simulink model "quadSim"  (R2019a)
settings: Solver=ode45  StartTime=0.0  StopTime=20  MaxStep=0.001  RelTol=1e-6  EnableMultiTasking=on
values from neighbouring files (symbols this model uses):
  bodyHalf = 0.3    [drone.m]
  hoverVel = trustPerPropeller / Ktrust    (= 50.511573882)    [drone.m]
  hoverVoltage = hoverCurrent * Ra + hoverRPM / Kv    (= 1.1)    [drone.m]
  KDrag = ampMax * Km / (rpmMax / 60 * 2 * pi)    (= 7.30185461146e-05)    [drone.m]    (also in propeller.m = 5.03149938834e-05)
  Km = 60/(Kv * 2 * pi)    (= 0.00536477336265)    [drone.m]    (also in propeller.m)
  Ktrust = (trustMax * g)/(rpmMax / 60 * 2 * pi)    (= 0.0427122505634)    [drone.m]    (also in propeller.m = 0.00501338070739)
  motorMass = 0.055    [drone.m]
  propellerMass = 0.015    [drone.m]
  Ra = RaVolt/ampMax    (= 1.20584269663)    [drone.m]    (also in propeller.m = 0.173442288049)
  s = tf('s')    [step-af-drone.m]
  Ts = 0.002    [drone.m]    (also in propeller.m)
undefined symbols (not defined in the file or in its folder): X, Y, Z
libraries: sm_lib x32, nesl_utility x23
(part 1 of 2)
settings Model: Creator=chr  LastModifiedBy=Hillerup
settings DataIOCC: LimitDataPoints=on  SaveFormat=Array  ReturnWorkspaceOutputs=off
settings OptimizationCC: LifeSpan=inf
settings DebuggingCC: SFUnexpectedBacktrackingDiag=warning  SFNoUnconditionalDefaultTransitionDiag=warning  SFExecutionAtInitializationDiag=none  ArithmeticOperatorsInVariantConditions=warning
settings HardwareCC: ProdBitPerPointer=32  ProdBitPerSizeT=32  ProdBitPerPtrDiffT=32  ProdLargestAtomicFloat=None  ProdIntDivRoundTo=Undefined  ProdEndianess=Unspecified  ProdWordSize=32  ProdHWDeviceType=32-bit Generic
settings ModelReferenceCC: PropagateSignalLabelsOutOfModel=off
settings SFSimCC: SimUseLocalCustomCode=off
settings RTWCC: RTWUseLocalCustomCode=off
settings CodeAppCC: StateflowObjectComments=on
settings GRTTargetCC: TargetLangStandard=C89/C90 (ANSI)  GeneratePreprocessorConditionals=Disable all
settings ConfigComp: CovMetricSettings=dw  CovHtmlReporting=on  CovSaveCumulativeToWorkspaceVar=on  CovSaveSingleToWorkspaceVar=on  CovExternalEMLEnable=off
settings SimscapeCC: SimscapeNormalizeSystem=off  SimscapeLogType=all  SimscapeLogDataHistory=10000
settings ConfigurationSet: Description=SimMechanics 2G

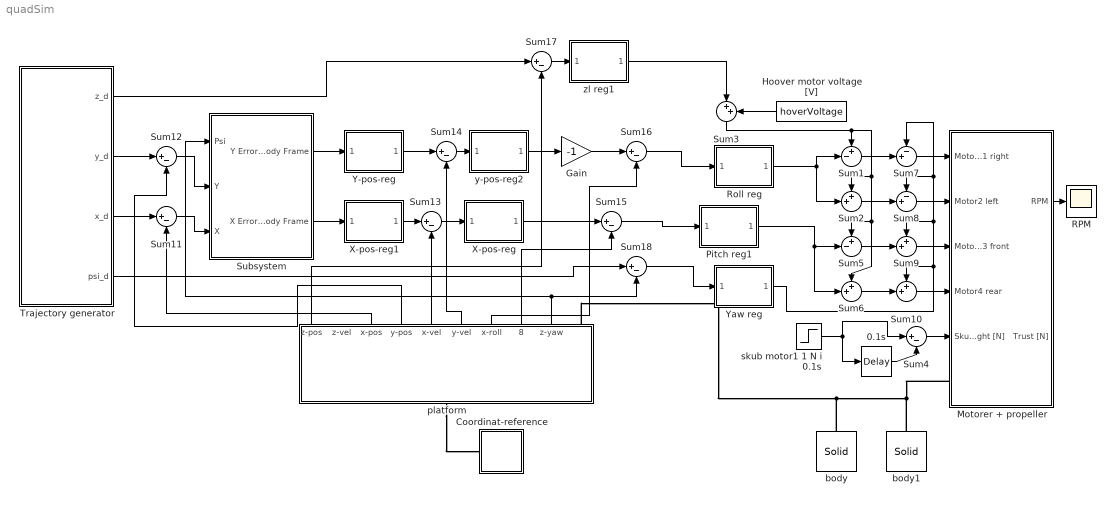
== system quadSim ==
  0.1s : TransportDelay  DelayTime=0.1
  Coordinat-reference : Subsystem
  Gain : Gain  Gain=-1
  Hoover motor voltage [V] : Constant  Value=hoverVoltage
  Motorer + propeller : Subsystem
  Pitch reg1 : Subsystem
  RPM : Scope
  Roll reg : Subsystem
  Subsystem : Subsystem
  Sum1 : Sum  Inputs=+-|
  Sum{2,6,9..10} (4 alike) : Sum  Inputs=++|
  Sum{4,11..18} (9 alike) : Sum  Inputs=|+-
  Sum3 : Sum  Inputs=|++
  Sum5 : Sum  Inputs=+-|
  Sum7 : Sum  Inputs=-+|
  Sum8 : Sum  Inputs=-+|
  Trajectory generator : Subsystem  TreatAsAtomicUnit=on
  X-pos-reg : Subsystem
  X-pos-reg1 : Subsystem
  Y-pos-reg : Subsystem
  "Yaw reg " : Subsystem
  body : sm_lib/Body Elements/Solid  InertiaType=CalculateFromGeometry  Mass=bodyHalf  MassUnits=kg  CenterOfMass=[0 0 0]  CenterOfMassUnits=m  MomentsOfInertia=[1 1 1]  MomentsOfInertiaUnits=kg*m^2  ProductsOfInertia=[0 0 0]  ProductsOfInertiaUnits=kg*m^2  BasedOnType=Mass  Density=1000  DensityUnits=kg/(m^3)  DoExposeReferenceFrame=on  SerializedFrames=<Frames/>  GraphicType=FromGeometry  MarkerShape=Sphere  MarkerSize=10  MarkerSizeUnits=m  GraphicVisPropType=SimpleVisualProperties  GraphicDiffuseColor=[0.5 0.5 0.5]  GraphicSpecularColor=[0.5 0.5 0.5 1.0]  GraphicAmbientColor=[0.15 0.15 0.15 1.0]  GraphicEmissiveColor=[0.0 0.0 0.0 1.0]  GraphicShininess=75  GraphicOpacity=1.0  GeometryShape=Brick  RectangleSize=[1 1]  RectangleSizeUnits=m  BrickDimensions=[0.04 0.4 0.03]  BrickDimensionUnits=m  CylinderRadius=0.02  CylinderRadiusUnits=m  CylinderLength=0.05  CylinderLengthUnits=m  SphereRadius=1  SphereRadiusUnits=m  EllipsoidRadii=[1 1 1]  EllipsoidRadiiUnits=m  ExtrusionCrossSection=[1 1; -1 1; -1 -1; 1 -1]  ExtrusionCrossSectionUnits=m  ExtrusionLength=1  ExtrusionLengthUnits=m  PolygonNumSides=3  PolygonOuterRadius=1  PolygonOuterRadiusUnits=m  ExtGeomFileType=STL  ExtGeomFileUnits=m  RevolutionCrossSection=[1 1; 1 -1; 2 -1; 2 1]  RevolutionCrossSectionUnits=m  RevolutionExtent=Full  RevolutionAngle=180  RevolutionAngleUnits=deg
  body1 : sm_lib/Body Elements/Solid  InertiaType=CalculateFromGeometry  Mass=bodyHalf  MassUnits=kg  CenterOfMass=[0 0 0]  CenterOfMassUnits=m  MomentsOfInertia=[1 1 1]  MomentsOfInertiaUnits=kg*m^2  ProductsOfInertia=[0 0 0]  ProductsOfInertiaUnits=kg*m^2  BasedOnType=Mass  Density=1000  DensityUnits=kg/(m^3)  DoExposeReferenceFrame=on  SerializedFrames=<Frames/>  GraphicType=FromGeometry  MarkerShape=Sphere  MarkerSize=10  MarkerSizeUnits=m  GraphicVisPropType=SimpleVisualProperties  GraphicDiffuseColor=[0.5 0.5 0.5]  GraphicSpecularColor=[0.5 0.5 0.5 1.0]  GraphicAmbientColor=[0.15 0.15 0.15 1.0]  GraphicEmissiveColor=[0.0 0.0 0.0 1.0]  GraphicShininess=75  GraphicOpacity=1.0  GeometryShape=Brick  RectangleSize=[1 1]  RectangleSizeUnits=m  BrickDimensions=[0.4 0.04 0.03]  BrickDimensionUnits=m  CylinderRadius=0.02  CylinderRadiusUnits=m  CylinderLength=0.05  CylinderLengthUnits=m  SphereRadius=1  SphereRadiusUnits=m  EllipsoidRadii=[1 1 1]  EllipsoidRadiiUnits=m  ExtrusionCrossSection=[1 1; -1 1; -1 -1; 1 -1]  ExtrusionCrossSectionUnits=m  ExtrusionLength=1  ExtrusionLengthUnits=m  PolygonNumSides=3  PolygonOuterRadius=1  PolygonOuterRadiusUnits=m  ExtGeomFileType=STL  ExtGeomFileUnits=m  RevolutionCrossSection=[1 1; 1 -1; 2 -1; 2 1]  RevolutionCrossSectionUnits=m  RevolutionExtent=Full  RevolutionAngle=180  RevolutionAngleUnits=deg
  platform : Subsystem
  skub motor1 1 N i 0.1s : Step  Time=2  SampleTime=0
  y-pos-reg2 : Subsystem
  zl reg1 : Subsystem
  wires:
  Motorer + propeller/1(RPM) -> RPM/1
  Sum3/1 -> Sum1/1, Sum6/1, Sum5/1, Sum2/1
  Sum4/1 -> Motorer + propeller/5(Skub right [N])
  Sum1/1 -> Sum7/2
  Sum2/1 -> Sum8/2
  Sum5/1 -> Sum9/2
  Sum6/1 -> Sum10/2
  Sum10/1 -> Motorer + propeller/4(Motor4 rear)
  Sum9/1 -> Motorer + propeller/3(Motor3 front)
  Sum8/1 -> Motorer + propeller/2(Motor2 left)
  Sum7/1 -> Motorer + propeller/1(Motor1 right)
  skub motor1 1 N i 0.1s/1 -> Sum4/1, 0.1s/1
  0.1s/1 -> Sum4/2
  platform/9(z-yaw) -> Sum18/2, Subsystem/1(Psi)
  Hoover motor voltage [V]/1 -> Sum3/2
  platform/3(x-pos) -> Sum11/2
  Trajectory generator/3(x_d) -> Sum11/1
  Sum11/1 -> Subsystem/3(X)
  Sum12/1 -> Subsystem/2(Y)
  Trajectory generator/2(y_d) -> Sum12/1
  zl reg1/1(u-roll) -> Sum3/1
  "Yaw reg "/1(u - yaw) -> Sum7/1, Sum8/1, Sum9/1, Sum10/1
  platform/7(x-roll) -> Sum16/2
  Sum17/1 -> zl reg1/1(error)
  Trajectory generator/1(z_d) -> Sum17/1
  platform/1(z-pos) -> Sum17/2
  Sum15/1 -> Pitch reg1/1(error)
  Sum18/1 -> "Yaw reg "/1(error)
  Trajectory generator/4(psi_d) -> Sum18/1
  platform/8(y-pitch) -> Sum15/2
  Subsystem/1(Y Error in Body Frame) -> Y-pos-reg/1(error_y)
  Subsystem/2(X Error in body Frame) -> X-pos-reg1/1(error_x)
  X-pos-reg1/1(u - pitch) -> Sum13/1
  Y-pos-reg/1(u - pitch) -> Sum14/1
  Roll reg/1(u-roll) -> Sum1/2, Sum2/2
  Pitch reg1/1(u-roll) -> Sum5/2, Sum6/2
  platform/4(y-pos) -> Sum12/2
  platform/5(x-vel) -> Sum13/2
  Sum13/1 -> X-pos-reg/1(error_x)
  Sum14/1 -> y-pos-reg2/1(error_x)
  y-pos-reg2/1(u - pitch) -> Gain/1
  X-pos-reg/1(u - pitch) -> Sum15/1
  platform/6(y-vel) -> Sum14/2
  Sum16/1 -> Roll reg/1(error)
  Gain/1 -> Sum16/1
  connections:
  platform/LConn1 -- Coordinat-reference/RConn1
  body/RConn1 -- body1/RConn1 -- Motorer + propeller/LConn1 -- platform/RConn1

== system quadSim/Coordinat-reference ==
  Mechanism Configuration : sm_lib/Utilities/Mechanism Configuration  UniformGravity=Constant  GravityVector=[0 0 -9.80665]  GravityUnits=m/s^2  LinearizationDelta=0.001
  Solver Configuration : nesl_utility/Solver Configuration  PhysicalDomain=network_engine_domain  SubClassName=solver  LeftPortType=input  RightPortType=generic  Tones=[]  Harmonics=[]  SimulateNoise=off  Profile=off  UseLocalSampling=off  EnableSwitchedLinearOptims=on  FrequencyDomain=off  UseCCode=off  RelTol=0.001  AbsTol=1e-06  MinStep=1e-09  ToWorkspace=off  RevertToSquareIcSolve=off  NumHomotopyIterations=100  PhasorMode=off  PhasorModeNumHarmonics=1  DoDC=off  ResidualTolerance=1e-09  UseLocalSolver=off  LocalSolverChoice=NE_BACKWARD_EULER_ADVANCER  LocalSolverSampleTime=0.001  DoFixedCost=off  MaxNonlinIter=3  MaxModeIter=2  LinearAlgebra=Sparse  EquationFormulation=NE_TIME_EF  DelaysMemoryBudget=1024  AutomaticFiltering=on  FilteringTimeConstant=0.001  PartitionStorageMethod=AS_NEEDED  PartitionMemoryBudget=1024  PartitionMethod=FAST
  World Frame : sm_lib/Frames and Transforms/World Frame
  ground : sm_lib/Body Elements/Solid  InertiaType=CalculateFromGeometry  Mass=1  MassUnits=kg  CenterOfMass=[0 0 0]  CenterOfMassUnits=m  MomentsOfInertia=[1 1 1]  MomentsOfInertiaUnits=kg*m^2  ProductsOfInertia=[0 0 0]  ProductsOfInertiaUnits=kg*m^2  BasedOnType=Mass  Density=1000  DensityUnits=kg/(m^3)  DoExposeReferenceFrame=on  SerializedFrames=<Frames/>  GraphicType=FromGeometry  MarkerShape=Sphere  MarkerSize=10  MarkerSizeUnits=m  GraphicVisPropType=SimpleVisualProperties  GraphicDiffuseColor=[0.2 0.5 0.2]  GraphicSpecularColor=[0.5 0.5 0.5 1.0]  GraphicAmbientColor=[0.15 0.15 0.15 1.0]  GraphicEmissiveColor=[0.0 0.0 0.0 1.0]  GraphicShininess=75  GraphicOpacity=1.0  GeometryShape=Brick  RectangleSize=[1 1]  RectangleSizeUnits=m  BrickDimensions=[1 1 0.01]  BrickDimensionUnits=m  CylinderRadius=1  CylinderRadiusUnits=m  CylinderLength=1  CylinderLengthUnits=m  SphereRadius=1  SphereRadiusUnits=m  EllipsoidRadii=[1 1 1]  EllipsoidRadiiUnits=m  ExtrusionCrossSection=[1 1; -1 1; -1 -1; 1 -1]  ExtrusionCrossSectionUnits=m  ExtrusionLength=1  ExtrusionLengthUnits=m  PolygonNumSides=3  PolygonOuterRadius=1  PolygonOuterRadiusUnits=m  ExtGeomFileType=STL  ExtGeomFileUnits=m  RevolutionCrossSection=[1 1; 1 -1; 2 -1; 2 1]  RevolutionCrossSectionUnits=m  RevolutionExtent=Full  RevolutionAngle=180  RevolutionAngleUnits=deg
  Conn1 : PMIOPort  Side=Right
  connections:
  Solver Configuration/RConn1 -- Conn1/RConn1 -- ground/RConn1 -- World Frame/RConn1 -- Mechanism Configuration/RConn1

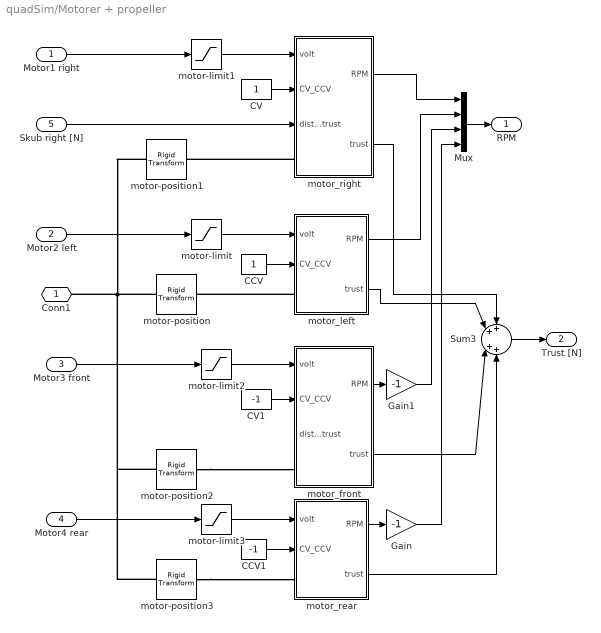
== system quadSim/Motorer + propeller ==
  Motor1 right : Inport
  Motor2 left : Inport  Port=2
  Motor3 front : Inport  Port=3
  Motor4 rear : Inport  Port=4
  Skub right [N] : Inport  Port=5
  CCV : Constant
  CCV1 : Constant  Value=-1
  CV : Constant
  CV1 : Constant  Value=-1
  Gain : Gain  Gain=-1
  Gain1 : Gain  Gain=-1
  Mux : Mux
  Sum3 : Sum  Inputs=++|++
  motor-limit{,1..3} (4 alike) : Saturate  UpperLimit=11  LowerLimit=0
  motor-position : sm_lib/Frames and Transforms/Rigid Transform  TranslationMethod=Cartesian  TranslationStandardOffset=0  TranslationLengthUnit=m  TranslationStandardAxis=+Z  TranslationCartesianOffset=[0 0.2 0.03]  TranslationROffset=0  TranslationROffsetUnits=m  TranslationZOffset=0  TranslationZOffsetUnits=m  TranslationThetaOffset=0  TranslationThetaOffsetUnits=deg  RotationMethod=StandardAxis  RotationAngleUnits=deg  RotationStandardAxis=+Y  RotationAngle=0.0  RotationArbitraryAxis=[0 0 1]  FollAlignAxisA=+X  BaseAlignAxisA=+Y  FollAlignAxisB=+Y  BaseAlignAxisB=+Z  RotationSequenceAxes=FollowerAxes  RotationSequence=XYX  RotationSequenceAngles=[0 0 0]  RotationSequenceAnglesUnits=deg  RotationMatrix=[1 0 0; 0 1 0; 0 0 1]
  motor-position1 : sm_lib/Frames and Transforms/Rigid Transform  TranslationMethod=Cartesian  TranslationStandardOffset=0  TranslationLengthUnit=m  TranslationStandardAxis=+Z  TranslationCartesianOffset=[0 -0.2 0.03]  TranslationROffset=0  TranslationROffsetUnits=m  TranslationZOffset=0  TranslationZOffsetUnits=m  TranslationThetaOffset=0  TranslationThetaOffsetUnits=deg  RotationMethod=StandardAxis  RotationAngleUnits=deg  RotationStandardAxis=+Y  RotationAngle=0.0  RotationArbitraryAxis=[0 0 1]  FollAlignAxisA=+X  BaseAlignAxisA=+Y  FollAlignAxisB=+Y  BaseAlignAxisB=+Z  RotationSequenceAxes=FollowerAxes  RotationSequence=XYX  RotationSequenceAngles=[0 0 0]  RotationSequenceAnglesUnits=deg  RotationMatrix=[1 0 0; 0 1 0; 0 0 1]
  motor-position2 : sm_lib/Frames and Transforms/Rigid Transform  TranslationMethod=Cartesian  TranslationStandardOffset=0  TranslationLengthUnit=m  TranslationStandardAxis=+Z  TranslationCartesianOffset=[0.2 0. 0.03]  TranslationROffset=0  TranslationROffsetUnits=m  TranslationZOffset=0  TranslationZOffsetUnits=m  TranslationThetaOffset=0  TranslationThetaOffsetUnits=deg  RotationMethod=StandardAxis  RotationAngleUnits=deg  RotationStandardAxis=+Y  RotationAngle=0.0  RotationArbitraryAxis=[0 0 1]  FollAlignAxisA=+X  BaseAlignAxisA=+Y  FollAlignAxisB=+Y  BaseAlignAxisB=+Z  RotationSequenceAxes=FollowerAxes  RotationSequence=XYX  RotationSequenceAngles=[0 0 0]  RotationSequenceAnglesUnits=deg  RotationMatrix=[1 0 0; 0 1 0; 0 0 1]
  motor-position3 : sm_lib/Frames and Transforms/Rigid Transform  TranslationMethod=Cartesian  TranslationStandardOffset=0  TranslationLengthUnit=m  TranslationStandardAxis=+Z  TranslationCartesianOffset=[-0.2 0. 0.03]  TranslationROffset=0  TranslationROffsetUnits=m  TranslationZOffset=0  TranslationZOffsetUnits=m  TranslationThetaOffset=0  TranslationThetaOffsetUnits=deg  RotationMethod=StandardAxis  RotationAngleUnits=deg  RotationStandardAxis=+Y  RotationAngle=0.0  RotationArbitraryAxis=[0 0 1]  FollAlignAxisA=+X  BaseAlignAxisA=+Y  FollAlignAxisB=+Y  BaseAlignAxisB=+Z  RotationSequenceAxes=FollowerAxes  RotationSequence=XYX  RotationSequenceAngles=[0 0 0]  RotationSequenceAnglesUnits=deg  RotationMatrix=[1 0 0; 0 1 0; 0 0 1]
  motor_front : Subsystem
  motor_left : Subsystem
  motor_rear : Subsystem
  motor_right : Subsystem
  Conn1 : PMIOPort  Side=Left
  RPM : Outport
  Trust [N] : Outport  Port=2
  wires:
  Motor1 right/1 -> motor-limit1/1
  Skub right [N]/1 -> motor_right/3(disturb_trust)
  motor_right/2(trust) -> Sum3/1
  motor_left/2(trust) -> Sum3/2
  CV/1 -> motor_right/2(CV_CCV)
  motor-limit1/1 -> motor_right/1(volt)
  CCV/1 -> motor_left/2(CV_CCV)
  Mux/1 -> RPM/1
  Sum3/1 -> Trust [N]/1
  Motor2 left/1 -> motor-limit/1
  motor-limit/1 -> motor_left/1(volt)
  motor_left/1(RPM) -> Mux/2
  Motor3 front/1 -> motor-limit2/1
  motor-limit2/1 -> motor_front/1(volt)
  Motor4 rear/1 -> motor-limit3/1
  motor-limit3/1 -> motor_rear/1(volt)
  CCV1/1 -> motor_rear/2(CV_CCV)
  CV1/1 -> motor_front/2(CV_CCV)
  motor_front/1(RPM) -> Gain1/1
  motor_rear/1(RPM) -> Gain/1
  motor_front/2(trust) -> Sum3/3
  motor_rear/2(trust) -> Sum3/4
  Gain1/1 -> Mux/3
  Gain/1 -> Mux/4
  motor_right/1(RPM) -> Mux/1
  connections:
  motor-position/LConn1 -- motor-position3/LConn1 -- motor-position2/LConn1 -- Conn1/RConn1 -- motor-position1/LConn1
  motor_right/LConn1 -- motor-position1/RConn1
  motor_left/LConn1 -- motor-position/RConn1
  motor-position2/RConn1 -- motor_front/LConn1
  motor-position3/RConn1 -- motor_rear/LConn1

== system quadSim/Pitch reg1 ==
  error : Inport
  KDr : Constant  Value=0.5
  KIr : Constant
  KPr : Constant  Value=0.8
  Roll-u : Scope
  roll-controller : Subsystem
  u-roll : Outport
  wires:
  KIr/1 -> roll-controller/1(KI)
  roll-controller/1(Out1) -> u-roll/1, Roll-u/1
  KPr/1 -> roll-controller/3(KP)
  KDr/1 -> roll-controller/2(KD)
  error/1 -> roll-controller/4(ref)

== system quadSim/Roll reg ==
  error : Inport
  KDr : Constant  Value=0.5
  KIr : Constant
  KPr : Constant  Value=0.8
  Roll-u : Scope
  roll-controller : Subsystem
  u-roll : Outport
  wires:
  KIr/1 -> roll-controller/1(KI)
  roll-controller/1(Out1) -> u-roll/1, Roll-u/1
  KPr/1 -> roll-controller/3(KP)
  KDr/1 -> roll-controller/2(KD)
  error/1 -> roll-controller/4(ref)

== system quadSim/Subsystem ==
  Psi : Inport
  Y : Inport  Port=2
  X : Inport  Port=3
  Product{,1..3} (4 alike) : Product
  Sum2 : Sum  Inputs=|++
  Sum4 : Sum  Inputs=|+-
  Trigonometric Functions : Trigonometry  Operator=sincos
  Y Error in Body Frame : Outport
  X Error in body Frame : Outport  Port=2
  wires:
  Trigonometric Functions/1 -> Product2/2, Product3/2  "sin(psi)"
  Product3/1 -> Sum4/2  "Xerr*sin(psi)"
  Sum2/1 -> X Error in body Frame/1  "Xerr*cos(psi)+Yerr*sin(psi)"
  Product1/1 -> Sum4/1  "Yerr*cos(psi)"
  Psi/1 -> Trigonometric Functions/1
  Product2/1 -> Sum2/2  "Yerr*sin(psi)"
  Trigonometric Functions/2 -> Product/2, Product1/2  "cos(psi)"
  Product/1 -> Sum2/1  "Xerr*cos(psi)"
  Sum4/1 -> Y Error in Body Frame/1  "Yerr*cos(psi)-Xerr*sin(psi)"
  Y/1 -> Product1/1, Product2/1  "Y Error"
  X/1 -> Product/1, Product3/1

== system quadSim/Trajectory generator ==
  Clock : Clock
      settings: Decimation=15
  Constant : Constant  Value=0
  Demux : Demux
  trajectory generator : MATLAB Function  TreatAsAtomicUnit=on
  z_d : Outport
  y_d : Outport  Port=2
  x_d : Outport  Port=3
  psi_d : Outport  Port=4
  wires:
  Clock/1 -> trajectory generator/1(t)
  trajectory generator/1(Cmd) -> Demux/1
  Demux/1 -> x_d/1
  Demux/2 -> y_d/1
  Demux/3 -> z_d/1
  Demux/4 -> psi_d/1
  Constant/1 -> trajectory generator/2(mode)

== system quadSim/X-pos-reg ==
  error_x : Inport
  KDr : Constant  Value=0.1
  KIr : Constant  Value=0
  KPr : Constant  Value=0.08
  Saturation : Saturate  UpperLimit=1  LowerLimit=-1
  X-pos-u : Scope
  x-pos-controller : Subsystem
  u - pitch : Outport
  wires:
  KIr/1 -> x-pos-controller/1(KI)
  x-pos-controller/1(Out1) -> Saturation/1
  KPr/1 -> x-pos-controller/3(KP)
  KDr/1 -> x-pos-controller/2(KD)
  error_x/1 -> x-pos-controller/4(error x)
  Saturation/1 -> u - pitch/1, X-pos-u/1

== system quadSim/X-pos-reg1 ==
  error_x : Inport
  KDr : Constant  Value=0.00015
  KIr : Constant  Value=0
  KPr : Constant
  Saturation : Saturate  UpperLimit=1  LowerLimit=-1
  X-pos-u : Scope
  x-pos-controller : Subsystem
  u - pitch : Outport
  wires:
  KIr/1 -> x-pos-controller/1(KI)
  x-pos-controller/1(Out1) -> Saturation/1
  KPr/1 -> x-pos-controller/3(KP)
  KDr/1 -> x-pos-controller/2(KD)
  error_x/1 -> x-pos-controller/4(error x)
  Saturation/1 -> u - pitch/1, X-pos-u/1

== system quadSim/Y-pos-reg ==
  error_y : Inport
  KDr : Constant  Value=0.00015
  KIr : Constant  Value=0
  KPr : Constant
  Saturation : Saturate  UpperLimit=1  LowerLimit=-1
  Y-pos-controller : Subsystem
  Y-pos-u : Scope
  u - pitch : Outport
  wires:
  Saturation/1 -> Y-pos-u/1, u - pitch/1
  error_y/1 -> Y-pos-controller/4(error_y)
  KDr/1 -> Y-pos-controller/2(KD)
  KPr/1 -> Y-pos-controller/3(KP)
  Y-pos-controller/1(Out1) -> Saturation/1
  KIr/1 -> Y-pos-controller/1(KI)

== system quadSim/Yaw reg  ==
  error : Inport
  KDr : Constant  Value=0.15
  KIr : Constant  Value=0
  KPr : Constant  Value=10
  Saturation : Saturate
  Yaw-controller : Subsystem
  Yaw-u : Scope
  u - yaw : Outport
  wires:
  KIr/1 -> Yaw-controller/1(KI)
  Yaw-controller/1(Out1) -> Saturation/1
  KPr/1 -> Yaw-controller/3(KP)
  KDr/1 -> Yaw-controller/2(KD)
  error/1 -> Yaw-controller/4(ref)
  Saturation/1 -> u - yaw/1, Yaw-u/1

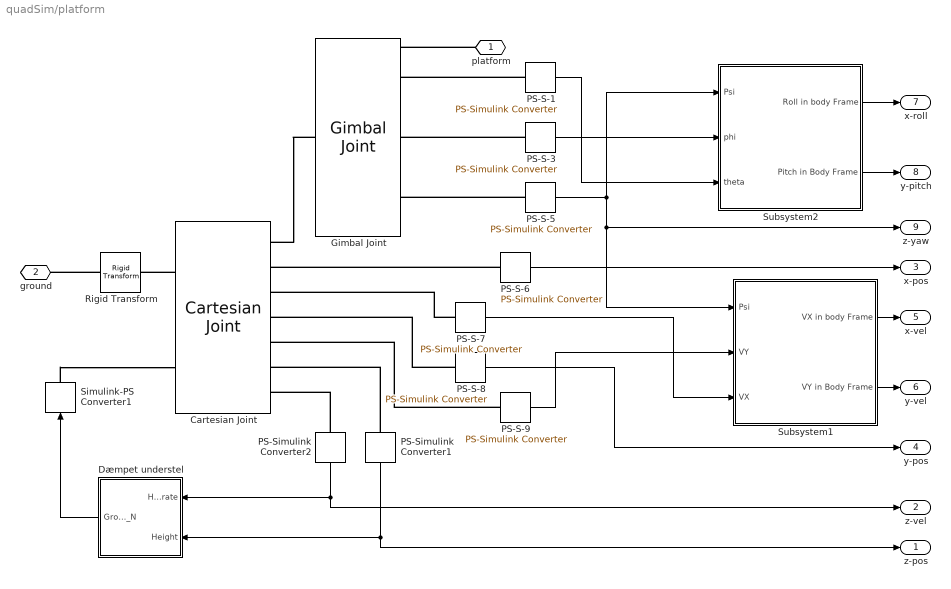
== system quadSim/platform ==
  Cartesian Joint : sm_lib/Joints/Cartesian Joint  SenseConstraintForce=off  SenseConstraintForceX=off  SenseConstraintForceY=off  SenseConstraintForceZ=off  SenseConstraintTorque=off  SenseConstraintTorqueX=off  SenseConstraintTorqueY=off  SenseConstraintTorqueZ=off  SenseTotalForce=off  SenseTotalForceX=off  SenseTotalForceY=off  SenseTotalForceZ=off  SenseTotalTorque=off  SenseTotalTorqueX=off  SenseTotalTorqueY=off  SenseTotalTorqueZ=off  CompositeWrenchDir=FollowerOnBase  CompositeWrenchFrame=BaseFrame  PxEquilibriumPosition=0  PxEquilibriumPositionUnits=m  PxSpringStiffness=0  PxSpringStiffnessUnits=N/m  PxDampingCoefficient=0  PxDampingCoefficientUnits=N/(m/s)  PxTorqueActuationMode=NoTorque  PxMotionActuationMode=ComputedMotion  PxSensePosition=on  PxSenseVelocity=on  PxSenseAcceleration=off  PxSenseTorqueForce=off  PxSenseLowerLimitTorqueForce=off  PxSenseUpperLimitTorqueForce=off  PxLowerLimitSpecify=off  PxLowerLimitBound=-1  PxLowerLimitBoundUnits=m  PxLowerLimitStiffness=1e6  PxLowerLimitStiffnessUnits=N/m  PxLowerLimitDamping=1e3  PxLowerLimitDampingUnits=N/(m/s)  PxLowerLimitTransitionRegionWidth=1e-4  PxLowerLimitTransitionRegionWidthUnits=m  PxUpperLimitSpecify=off  PxUpperLimitBound=1  PxUpperLimitBoundUnits=m  PxUpperLimitStiffness=1e6  PxUpperLimitStiffnessUnits=N/m  PxUpperLimitDamping=1e3  PxUpperLimitDampingUnits=N/(m/s)  PxUpperLimitTransitionRegionWidth=1e-4  PxUpperLimitTransitionRegionWidthUnits=m  PxPositionTargetSpecify=off  PxPositionTargetPriority=High  PxPositionTargetValue=0  PxPositionTargetValueUnits=m  PxVelocityTargetSpecify=off  PxVelocityTargetPriority=High  PxVelocityTargetValue=0  PxVelocityTargetValueUnits=m/s  PyEquilibriumPosition=0  PyEquilibriumPositionUnits=m  PySpringStiffness=0  PySpringStiffnessUnits=N/m  PyDampingCoefficient=0  PyDampingCoefficientUnits=N/(m/s)  PyTorqueActuationMode=NoTorque  PyMotionActuationMode=ComputedMotion  PySensePosition=on  PySenseVelocity=on  PySenseAcceleration=off  PySenseTorqueForce=off  PySenseLowerLimitTorqueForce=off  PySenseUpperLimitTorqueForce=off  PyLowerLimitSpecify=off  PyLowerLimitBound=-1  PyLowerLimitBoundUnits=m  PyLowerLimitStiffness=1e6  PyLowerLimitStiffnessUnits=N/m  PyLowerLimitDamping=1e3  PyLowerLimitDampingUnits=N/(m/s)  PyLowerLimitTransitionRegionWidth=1e-4  PyLowerLimitTransitionRegionWidthUnits=m  PyUpperLimitSpecify=off  PyUpperLimitBound=1  PyUpperLimitBoundUnits=m  PyUpperLimitStiffness=1e6  PyUpperLimitStiffnessUnits=N/m  PyUpperLimitDamping=1e3  PyUpperLimitDampingUnits=N/(m/s)  PyUpperLimitTransitionRegionWidth=1e-4  PyUpperLimitTransitionRegionWidthUnits=m  PyPositionTargetSpecify=off  PyPositionTargetPriority=High  PyPositionTargetValue=0  PyPositionTargetValueUnits=m  PyVelocityTargetSpecify=off  PyVelocityTargetPriority=High  PyVelocityTargetValue=0  PyVelocityTargetValueUnits=m/s  PzEquilibriumPosition=0  PzEquilibriumPositionUnits=m  PzSpringStiffness=0  PzSpringStiffnessUnits=N/m  PzDampingCoefficient=0  PzDampingCoefficientUnits=N/(m/s)  PzTorqueActuationMode=InputTorque  PzMotionActuationMode=ComputedMotion  PzSensePosition=on  PzSenseVelocity=on  PzSenseAcceleration=off  PzSenseTorqueForce=off  PzSenseLowerLimitTorqueForce=off  PzSenseUpperLimitTorqueForce=off  PzLowerLimitSpecify=off  PzLowerLimitBound=-1  PzLowerLimitBoundUnits=m  PzLowerLimitStiffness=1e6  PzLowerLimitStiffnessUnits=N/m  PzLowerLimitDamping=1e3  PzLowerLimitDampingUnits=N/(m/s)  PzLowerLimitTransitionRegionWidth=1e-4  PzLowerLimitTransitionRegionWidthUnits=m  PzUpperLimitSpecify=off  PzUpperLimitBound=1  PzUpperLimitBoundUnits=m  PzUpperLimitStiffness=1e6  PzUpperLimitStiffnessUnits=N/m  PzUpperLimitDamping=1e3  PzUpperLimitDampingUnits=N/(m/s)  PzUpperLimitTransitionRegionWidth=1e-4  PzUpperLimitTransitionRegionWidthUnits=m  PzPositionTargetSpecify=on  PzPositionTargetPriority=High  PzPositionTargetValue=1  PzPositionTargetValueUnits=m  PzVelocityTargetSpecify=off  PzVelocityTargetPriority=High  PzVelocityTargetValue=0  PzVelocityTargetValueUnits=m/s
  Dæmpet understel : Subsystem
  Gimbal Joint : sm_lib/Joints/Gimbal Joint  SenseConstraintForce=off  SenseConstraintForceX=off  SenseConstraintForceY=off  SenseConstraintForceZ=off  SenseConstraintTorque=off  SenseConstraintTorqueX=off  SenseConstraintTorqueY=off  SenseConstraintTorqueZ=off  SenseTotalForce=off  SenseTotalForceX=off  SenseTotalForceY=off  SenseTotalForceZ=off  SenseTotalTorque=off  SenseTotalTorqueX=off  SenseTotalTorqueY=off  SenseTotalTorqueZ=off  CompositeWrenchDir=FollowerOnBase  CompositeWrenchFrame=BaseFrame  RxEquilibriumPosition=0  RxEquilibriumPositionUnits=deg  RxSpringStiffness=0  RxSpringStiffnessUnits=N*m/deg  RxDampingCoefficient=0  RxDampingCoefficientUnits=N*m/(deg/s)  RxTorqueActuationMode=NoTorque  RxMotionActuationMode=ComputedMotion  RxSensePosition=on  RxSenseVelocity=on  RxSenseAcceleration=off  RxSenseTorqueForce=off  RxSenseLowerLimitTorqueForce=off  RxSenseUpperLimitTorqueForce=off  RxLowerLimitSpecify=off  RxLowerLimitBound=-90  RxLowerLimitBoundUnits=deg  RxLowerLimitStiffness=1e4  RxLowerLimitStiffnessUnits=N*m/deg  RxLowerLimitDamping=10  RxLowerLimitDampingUnits=N*m/(deg/s)  RxLowerLimitTransitionRegionWidth=0.1  RxLowerLimitTransitionRegionWidthUnits=deg  RxUpperLimitSpecify=off  RxUpperLimitBound=90  RxUpperLimitBoundUnits=deg  RxUpperLimitStiffness=1e4  RxUpperLimitStiffnessUnits=N*m/deg  RxUpperLimitDamping=10  RxUpperLimitDampingUnits=N*m/(deg/s)  RxUpperLimitTransitionRegionWidth=0.1  RxUpperLimitTransitionRegionWidthUnits=deg  RxPositionTargetSpecify=off  RxPositionTargetPriority=High  RxPositionTargetValue=0  RxPositionTargetValueUnits=deg  RxVelocityTargetSpecify=off  RxVelocityTargetPriority=High  RxVelocityTargetValue=0  RxVelocityTargetValueUnits=deg/s  RyEquilibriumPosition=0  RyEquilibriumPositionUnits=deg  RySpringStiffness=0  RySpringStiffnessUnits=N*m/deg  RyDampingCoefficient=0  RyDampingCoefficientUnits=N*m/(deg/s)  RyTorqueActuationMode=NoTorque  RyMotionActuationMode=ComputedMotion  RySensePosition=on  RySenseVelocity=on  RySenseAcceleration=off  RySenseTorqueForce=off  RySenseLowerLimitTorqueForce=off  RySenseUpperLimitTorqueForce=off  RyLowerLimitSpecify=off  RyLowerLimitBound=-90  RyLowerLimitBoundUnits=deg  RyLowerLimitStiffness=1e4  RyLowerLimitStiffnessUnits=N*m/deg  RyLowerLimitDamping=10  RyLowerLimitDampingUnits=N*m/(deg/s)  RyLowerLimitTransitionRegionWidth=0.1  RyLowerLimitTransitionRegionWidthUnits=deg  RyUpperLimitSpecify=off  RyUpperLimitBound=90  RyUpperLimitBoundUnits=deg  RyUpperLimitStiffness=1e4  RyUpperLimitStiffnessUnits=N*m/deg  RyUpperLimitDamping=10  RyUpperLimitDampingUnits=N*m/(deg/s)  RyUpperLimitTransitionRegionWidth=0.1  RyUpperLimitTransitionRegionWidthUnits=deg  RyPositionTargetSpecify=off  RyPositionTargetPriority=High  RyPositionTargetValue=0  RyPositionTargetValueUnits=deg  RyVelocityTargetSpecify=off  RyVelocityTargetPriority=High  RyVelocityTargetValue=0  RyVelocityTargetValueUnits=deg/s  RzEquilibriumPosition=0  RzEquilibriumPositionUnits=deg  RzSpringStiffness=0  RzSpringStiffnessUnits=N*m/deg  RzDampingCoefficient=0  RzDampingCoefficientUnits=N*m/(deg/s)  RzTorqueActuationMode=NoTorque  RzMotionActuationMode=ComputedMotion  RzSensePosition=on  RzSenseVelocity=on  RzSenseAcceleration=off  RzSenseTorqueForce=off  RzSenseLowerLimitTorqueForce=off  RzSenseUpperLimitTorqueForce=off  RzLowerLimitSpecify=off  RzLowerLimitBound=-90  RzLowerLimitBoundUnits=deg  RzLowerLimitStiffness=1e4  RzLowerLimitStiffnessUnits=N*m/deg  RzLowerLimitDamping=10  RzLowerLimitDampingUnits=N*m/(deg/s)  RzLowerLimitTransitionRegionWidth=0.1  RzLowerLimitTransitionRegionWidthUnits=deg  RzUpperLimitSpecify=off  RzUpperLimitBound=90  RzUpperLimitBoundUnits=deg  RzUpperLimitStiffness=1e4  RzUpperLimitStiffnessUnits=N*m/deg  RzUpperLimitDamping=10  RzUpperLimitDampingUnits=N*m/(deg/s)  RzUpperLimitTransitionRegionWidth=0.1  RzUpperLimitTransitionRegionWidthUnits=deg  RzPositionTargetSpecify=off  RzPositionTargetPriority=High  RzPositionTargetValue=0  RzPositionTargetValueUnits=deg  RzVelocityTargetSpecify=off  RzVelocityTargetPriority=High  RzVelocityTargetValue=0  RzVelocityTargetValueUnits=deg/s
      settings: SourceProductName=Simscape Multibody
  PS-S-{1,3,5..9} (7 alike) : nesl_utility/PS-Simulink Converter  PhysicalDomain=network_engine_domain  SubClassName=ps_output  LeftPortType=input  RightPortType=output  PseudoPeriodic=off  Frequencies=[]  Unit=1  AffineConversion=off
  PS-Simulink Converter1 : nesl_utility/PS-Simulink Converter  PhysicalDomain=network_engine_domain  SubClassName=ps_output  LeftPortType=input  RightPortType=output  PseudoPeriodic=off  Frequencies=[]  Unit=1  AffineConversion=off
  PS-Simulink Converter2 : nesl_utility/PS-Simulink Converter  PhysicalDomain=network_engine_domain  SubClassName=ps_output  LeftPortType=input  RightPortType=output  PseudoPeriodic=off  Frequencies=[]  Unit=1  AffineConversion=off
  Rigid Transform : sm_lib/Frames and Transforms/Rigid Transform  TranslationMethod=Cartesian  TranslationStandardOffset=0  TranslationLengthUnit=m  TranslationStandardAxis=+Z  TranslationCartesianOffset=[0 0 0.05]  TranslationROffset=0  TranslationROffsetUnits=m  TranslationZOffset=0  TranslationZOffsetUnits=m  TranslationThetaOffset=0  TranslationThetaOffsetUnits=deg  RotationMethod=StandardAxis  RotationAngleUnits=deg  RotationStandardAxis=+Z  RotationAngle=0.0  RotationArbitraryAxis=[0 0 1]  FollAlignAxisA=+X  BaseAlignAxisA=+Y  FollAlignAxisB=+Y  BaseAlignAxisB=+Z  RotationSequenceAxes=FollowerAxes  RotationSequence=XYX  RotationSequenceAngles=[0 0 0]  RotationSequenceAnglesUnits=deg  RotationMatrix=[1 0 0; 0 1 0; 0 0 1]
  Simulink-PS Converter1 : nesl_utility/Simulink-PS Converter  PhysicalDomain=network_engine_domain  SubClassName=ps_input  LeftPortType=input  RightPortType=output  PseudoPeriodic=off  Frequencies=[]  NoiseDistribution=none  NoiseParameters=[]  Unit=1  AffineConversion=off  FilteringAndDerivatives=zero  SimscapeFilterOrder=1  InputFilterTimeConstant=0.001  UdotUserProvided=1
  Subsystem1 : Subsystem
  Subsystem2 : Subsystem
  platform : PMIOPort  Side=Right
  ground : PMIOPort  Port=2  Side=Left
  z-pos : Outport
  z-vel : Outport  Port=2
  x-pos : Outport  Port=3
  y-pos : Outport  Port=4
  x-vel : Outport  Port=5
  y-vel : Outport  Port=6
  x-roll : Outport  Port=7
  y-pitch : Outport  Port=8
  z-yaw : Outport  Port=9
  wires:
  Dæmpet understel/1(Ground_N) -> Simulink-PS Converter1/1
  PS-Simulink Converter1/1 -> z-pos/1, Dæmpet understel/2(Height)
  PS-Simulink Converter2/1 -> Dæmpet understel/1(Heingt_rate), z-vel/1
  PS-S-6/1 -> x-pos/1
  PS-S-8/1 -> y-pos/1
  PS-S-5/1 -> z-yaw/1, Subsystem1/1(Psi), Subsystem2/1(Psi)
  Subsystem2/1(Roll in body Frame) -> x-roll/1
  PS-S-1/1 -> Subsystem2/3(theta)
  Subsystem2/2(Pitch in Body Frame) -> y-pitch/1
  PS-S-3/1 -> Subsystem2/2(phi)
  Subsystem1/1(VX in body Frame) -> x-vel/1
  PS-S-7/1 -> Subsystem1/3(VX)
  Subsystem1/2(VY in Body Frame) -> y-vel/1
  PS-S-9/1 -> Subsystem1/2(VY)
  connections:
  Rigid Transform/LConn1 -- ground/RConn1
  Simulink-PS Converter1/RConn1 -- Cartesian Joint/LConn2
  PS-Simulink Converter1/LConn1 -- Cartesian Joint/RConn6
  PS-Simulink Converter2/LConn1 -- Cartesian Joint/RConn7
  platform/RConn1 -- Gimbal Joint/RConn1
  PS-S-6/LConn1 -- Cartesian Joint/RConn2
  PS-S-7/LConn1 -- Cartesian Joint/RConn3
  PS-S-8/LConn1 -- Cartesian Joint/RConn4
  PS-S-9/LConn1 -- Cartesian Joint/RConn5
  Cartesian Joint/LConn1 -- Rigid Transform/RConn1
  Gimbal Joint/LConn1 -- Cartesian Joint/RConn1
  PS-S-1/LConn1 -- Gimbal Joint/RConn2
  PS-S-3/LConn1 -- Gimbal Joint/RConn4
  PS-S-5/LConn1 -- Gimbal Joint/RConn6

== system quadSim/y-pos-reg2 ==
  error_x : Inport
  KDr : Constant  Value=0.1
  KIr : Constant  Value=0
  KPr : Constant  Value=0.08
  Saturation : Saturate  UpperLimit=1  LowerLimit=-1
  X-pos-u : Scope
  x-pos-controller : Subsystem
  u - pitch : Outport
  wires:
  KIr/1 -> x-pos-controller/1(KI)
  x-pos-controller/1(Out1) -> Saturation/1
  KPr/1 -> x-pos-controller/3(KP)
  KDr/1 -> x-pos-controller/2(KD)
  error_x/1 -> x-pos-controller/4(error x)
  Saturation/1 -> u - pitch/1, X-pos-u/1

== system quadSim/zl reg1 ==
  error : Inport
  KDr : Constant  Value=0.8
  KIr : Constant  Value=0.7
  KPr : Constant  Value=3
  Roll-u : Scope
  roll-controller : Subsystem
  u-roll : Outport
  wires:
  KIr/1 -> roll-controller/1(KI)
  roll-controller/1(Out1) -> u-roll/1, Roll-u/1
  KPr/1 -> roll-controller/3(KP)
  KDr/1 -> roll-controller/2(KD)
  error/1 -> roll-controller/4(ref)

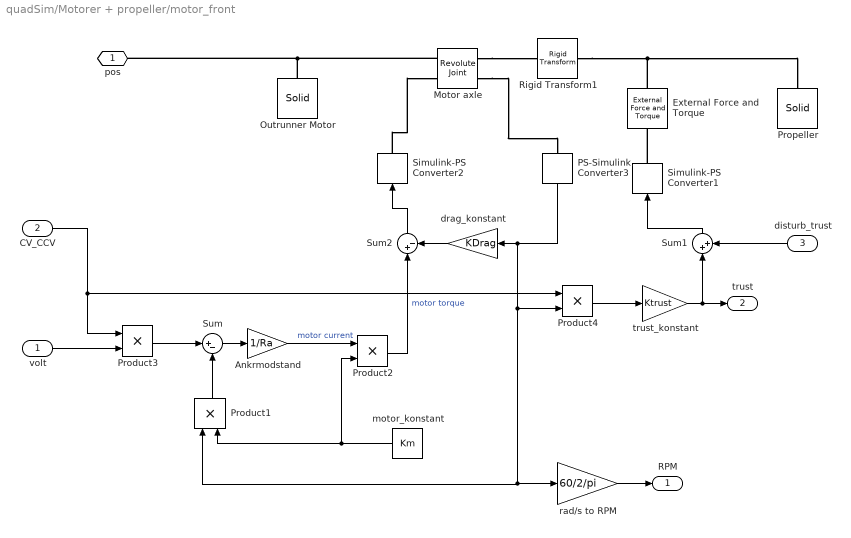
== system quadSim/Motorer + propeller/motor_front ==
  volt : Inport
  CV_CCV : Inport  Port=2
  disturb_trust : Inport  Port=3
  Ankrmodstand : Gain  Gain=1/Ra
  External Force and Torque : sm_lib/Forces and Torques/External Force and Torque  ForceResolutionFrame=AttachedFrame  EnableForceX=off  EnableForceY=off  EnableForceZ=on  EnableForce=off  TorqueResolutionFrame=AttachedFrame  EnableTorqueX=off  EnableTorqueY=off  EnableTorqueZ=off  EnableTorque=off
  Motor axle : sm_lib/Joints/Revolute Joint  SenseConstraintForce=off  SenseConstraintForceX=off  SenseConstraintForceY=off  SenseConstraintForceZ=off  SenseConstraintTorque=off  SenseConstraintTorqueX=off  SenseConstraintTorqueY=off  SenseConstraintTorqueZ=off  SenseTotalForce=off  SenseTotalForceX=off  SenseTotalForceY=off  SenseTotalForceZ=off  SenseTotalTorque=off  SenseTotalTorqueX=off  SenseTotalTorqueY=off  SenseTotalTorqueZ=off  CompositeWrenchDir=FollowerOnBase  CompositeWrenchFrame=BaseFrame  EquilibriumPosition=0  EquilibriumPositionUnits=deg  SpringStiffness=0  SpringStiffnessUnits=N*m/deg  DampingCoefficient=0  DampingCoefficientUnits=N*m/(deg/s)  TorqueActuationMode=InputTorque  MotionActuationMode=ComputedMotion  SensePosition=off  SenseVelocity=on  SenseAcceleration=off  SenseTorqueForce=off  SenseLowerLimitTorqueForce=off  SenseUpperLimitTorqueForce=off  LowerLimitSpecify=off  LowerLimitBound=-90  LowerLimitBoundUnits=deg  LowerLimitStiffness=1e4  LowerLimitStiffnessUnits=N*m/deg  LowerLimitDamping=10  LowerLimitDampingUnits=N*m/(deg/s)  LowerLimitTransitionRegionWidth=0.1  LowerLimitTransitionRegionWidthUnits=deg  UpperLimitSpecify=off  UpperLimitBound=90  UpperLimitBoundUnits=deg  UpperLimitStiffness=1e4  UpperLimitStiffnessUnits=N*m/deg  UpperLimitDamping=10  UpperLimitDampingUnits=N*m/(deg/s)  UpperLimitTransitionRegionWidth=0.1  UpperLimitTransitionRegionWidthUnits=deg  PositionTargetSpecify=off  PositionTargetPriority=High  PositionTargetValue=0  PositionTargetValueUnits=deg  VelocityTargetSpecify=on  VelocityTargetPriority=High  VelocityTargetValue=-hoverVel  VelocityTargetValueUnits=rad/s
  Outrunner Motor : sm_lib/Body Elements/Solid  InertiaType=CalculateFromGeometry  Mass=motorMass  MassUnits=kg  CenterOfMass=[0 0 0]  CenterOfMassUnits=m  MomentsOfInertia=[1 1 1]  MomentsOfInertiaUnits=kg*m^2  ProductsOfInertia=[0 0 0]  ProductsOfInertiaUnits=kg*m^2  BasedOnType=Mass  Density=1000  DensityUnits=kg/(m^3)  DoExposeReferenceFrame=on  SerializedFrames=<Frames/>  GraphicType=FromGeometry  MarkerShape=Sphere  MarkerSize=10  MarkerSizeUnits=m  GraphicVisPropType=SimpleVisualProperties  GraphicDiffuseColor=[1.0 0.8 0.0]  GraphicSpecularColor=[0.5 0.5 0.5 1.0]  GraphicAmbientColor=[0.15 0.15 0.15 1.0]  GraphicEmissiveColor=[0.0 0.0 0.0 1.0]  GraphicShininess=75  GraphicOpacity=1.0  GeometryShape=Cylinder  RectangleSize=[1 1]  RectangleSizeUnits=m  BrickDimensions=[1 1 0.01]  BrickDimensionUnits=m  CylinderRadius=0.02  CylinderRadiusUnits=m  CylinderLength=0.05  CylinderLengthUnits=m  SphereRadius=1  SphereRadiusUnits=m  EllipsoidRadii=[1 1 1]  EllipsoidRadiiUnits=m  ExtrusionCrossSection=[1 1; -1 1; -1 -1; 1 -1]  ExtrusionCrossSectionUnits=m  ExtrusionLength=1  ExtrusionLengthUnits=m  PolygonNumSides=3  PolygonOuterRadius=1  PolygonOuterRadiusUnits=m  ExtGeomFileType=STL  ExtGeomFileUnits=m  RevolutionCrossSection=[1 1; 1 -1; 2 -1; 2 1]  RevolutionCrossSectionUnits=m  RevolutionExtent=Full  RevolutionAngle=180  RevolutionAngleUnits=deg
  PS-Simulink Converter3 : nesl_utility/PS-Simulink Converter  PhysicalDomain=network_engine_domain  SubClassName=ps_output  LeftPortType=input  RightPortType=output  PseudoPeriodic=off  Frequencies=[]  Unit=1  AffineConversion=off
  Product{1..4} (4 alike) : Product
  Propeller : sm_lib/Body Elements/Solid  InertiaType=CalculateFromGeometry  Mass=propellerMass  MassUnits=kg  CenterOfMass=[0 0 0]  CenterOfMassUnits=m  MomentsOfInertia=[1 1 1]  MomentsOfInertiaUnits=kg*m^2  ProductsOfInertia=[0 0 0]  ProductsOfInertiaUnits=kg*m^2  BasedOnType=Mass  Density=1000  DensityUnits=kg/(m^3)  DoExposeReferenceFrame=on  SerializedFrames=<Frames/>  GraphicType=FromGeometry  MarkerShape=Sphere  MarkerSize=10  MarkerSizeUnits=m  GraphicVisPropType=SimpleVisualProperties  GraphicDiffuseColor=[1.0 0.8 0.0]  GraphicSpecularColor=[0.5 0.5 0.5 1.0]  GraphicAmbientColor=[0.15 0.15 0.15 1.0]  GraphicEmissiveColor=[0.0 0.0 0.0 1.0]  GraphicShininess=75  GraphicOpacity=1.0  GeometryShape=Brick  RectangleSize=[1 1]  RectangleSizeUnits=m  BrickDimensions=[0.2 0.03 0.01]  BrickDimensionUnits=m  CylinderRadius=0.02  CylinderRadiusUnits=m  CylinderLength=0.05  CylinderLengthUnits=m  SphereRadius=1  SphereRadiusUnits=m  EllipsoidRadii=[1 1 1]  EllipsoidRadiiUnits=m  ExtrusionCrossSection=[1 1; -1 1; -1 -1; 1 -1]  ExtrusionCrossSectionUnits=m  ExtrusionLength=1  ExtrusionLengthUnits=m  PolygonNumSides=3  PolygonOuterRadius=1  PolygonOuterRadiusUnits=m  ExtGeomFileType=STL  ExtGeomFileUnits=m  RevolutionCrossSection=[1 1; 1 -1; 2 -1; 2 1]  RevolutionCrossSectionUnits=m  RevolutionExtent=Full  RevolutionAngle=180  RevolutionAngleUnits=deg
  Rigid Transform1 : sm_lib/Frames and Transforms/Rigid Transform  TranslationMethod=Cartesian  TranslationStandardOffset=0  TranslationLengthUnit=m  TranslationStandardAxis=+Z  TranslationCartesianOffset=[0 0 0.03]  TranslationROffset=0  TranslationROffsetUnits=m  TranslationZOffset=0  TranslationZOffsetUnits=m  TranslationThetaOffset=0  TranslationThetaOffsetUnits=deg  RotationMethod=StandardAxis  RotationAngleUnits=deg  RotationStandardAxis=+Z  RotationAngle=0.0  RotationArbitraryAxis=[0 0 1]  FollAlignAxisA=+X  BaseAlignAxisA=+Y  FollAlignAxisB=+Y  BaseAlignAxisB=+Z  RotationSequenceAxes=FollowerAxes  RotationSequence=XYX  RotationSequenceAngles=[0 0 0]  RotationSequenceAnglesUnits=deg  RotationMatrix=[1 0 0; 0 1 0; 0 0 1]
  Simulink-PS Converter1 : nesl_utility/Simulink-PS Converter  PhysicalDomain=network_engine_domain  SubClassName=ps_input  LeftPortType=input  RightPortType=output  PseudoPeriodic=off  Frequencies=[]  NoiseDistribution=none  NoiseParameters=[]  Unit=1  AffineConversion=off  FilteringAndDerivatives=zero  SimscapeFilterOrder=1  InputFilterTimeConstant=0.001  UdotUserProvided=1
  Simulink-PS Converter2 : nesl_utility/Simulink-PS Converter  PhysicalDomain=network_engine_domain  SubClassName=ps_input  LeftPortType=input  RightPortType=output  PseudoPeriodic=off  Frequencies=[]  NoiseDistribution=none  NoiseParameters=[]  Unit=1  AffineConversion=off  FilteringAndDerivatives=zero  SimscapeFilterOrder=1  InputFilterTimeConstant=0.001  UdotUserProvided=1
  Sum : Sum  Inputs=|+-
  Sum1 : Sum  Inputs=|++
  Sum2 : Sum  Inputs=|+-
  drag_konstant : Gain  Gain=KDrag
  motor_konstant : Constant  Value=Km
  rad/s to RPM : Gain  Gain=60/2/pi
  trust_konstant : Gain  Gain=Ktrust
  pos : PMIOPort  Side=Left
  RPM : Outport
  trust : Outport  Port=2
  wires:
  disturb_trust/1 -> Sum1/2
  Sum1/1 -> Simulink-PS Converter1/1
  Product4/1 -> trust_konstant/1
  CV_CCV/1 -> Product4/1, Product3/1
  Product3/1 -> Sum/1
  volt/1 -> Product3/2
  drag_konstant/1 -> Sum2/2
  Sum2/1 -> Simulink-PS Converter2/1
  PS-Simulink Converter3/1 -> Product4/2, Product1/1, rad/s to RPM/1, drag_konstant/1
  Sum/1 -> Ankrmodstand/1
  Ankrmodstand/1 -> Product2/1  "motor current"
  Product2/1 -> Sum2/1  "motor torque"
  trust_konstant/1 -> trust/1, Sum1/1
  Product1/1 -> Sum/2
  motor_konstant/1 -> Product1/2, Product2/2
  rad/s to RPM/1 -> RPM/1
  connections:
  Rigid Transform1/RConn1 -- External Force and Torque/RConn1 -- Propeller/RConn1
  Outrunner Motor/RConn1 -- pos/RConn1 -- Motor axle/LConn1
  Simulink-PS Converter2/RConn1 -- Motor axle/LConn2
  Motor axle/RConn1 -- Rigid Transform1/LConn1
  Motor axle/RConn2 -- PS-Simulink Converter3/LConn1
  Simulink-PS Converter1/RConn1 -- External Force and Torque/LConn1

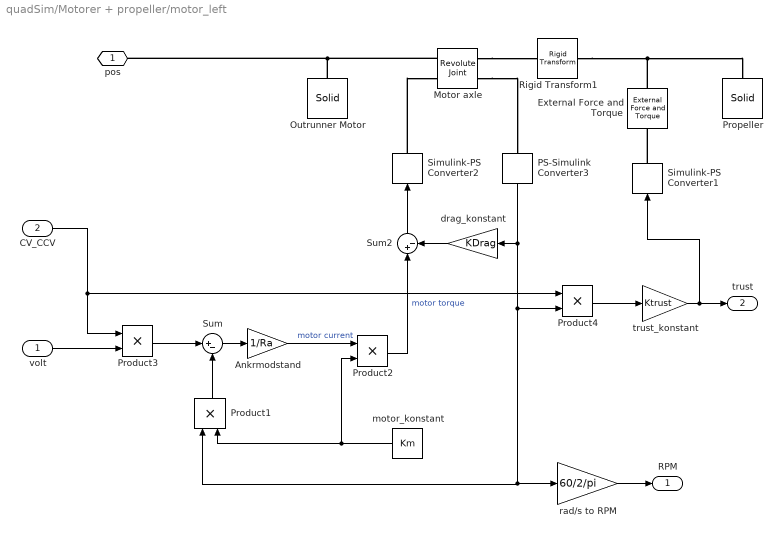
== system quadSim/Motorer + propeller/motor_left ==
  volt : Inport
  CV_CCV : Inport  Port=2
  Ankrmodstand : Gain  Gain=1/Ra
  External Force and Torque : sm_lib/Forces and Torques/External Force and Torque  ForceResolutionFrame=AttachedFrame  EnableForceX=off  EnableForceY=off  EnableForceZ=on  EnableForce=off  TorqueResolutionFrame=AttachedFrame  EnableTorqueX=off  EnableTorqueY=off  EnableTorqueZ=off  EnableTorque=off
  Motor axle : sm_lib/Joints/Revolute Joint  SenseConstraintForce=off  SenseConstraintForceX=off  SenseConstraintForceY=off  SenseConstraintForceZ=off  SenseConstraintTorque=off  SenseConstraintTorqueX=off  SenseConstraintTorqueY=off  SenseConstraintTorqueZ=off  SenseTotalForce=off  SenseTotalForceX=off  SenseTotalForceY=off  SenseTotalForceZ=off  SenseTotalTorque=off  SenseTotalTorqueX=off  SenseTotalTorqueY=off  SenseTotalTorqueZ=off  CompositeWrenchDir=FollowerOnBase  CompositeWrenchFrame=BaseFrame  EquilibriumPosition=0  EquilibriumPositionUnits=deg  SpringStiffness=0  SpringStiffnessUnits=N*m/deg  DampingCoefficient=0  DampingCoefficientUnits=N*m/(deg/s)  TorqueActuationMode=InputTorque  MotionActuationMode=ComputedMotion  SensePosition=off  SenseVelocity=on  SenseAcceleration=off  SenseTorqueForce=off  SenseLowerLimitTorqueForce=off  SenseUpperLimitTorqueForce=off  LowerLimitSpecify=off  LowerLimitBound=-90  LowerLimitBoundUnits=deg  LowerLimitStiffness=1e4  LowerLimitStiffnessUnits=N*m/deg  LowerLimitDamping=10  LowerLimitDampingUnits=N*m/(deg/s)  LowerLimitTransitionRegionWidth=0.1  LowerLimitTransitionRegionWidthUnits=deg  UpperLimitSpecify=off  UpperLimitBound=90  UpperLimitBoundUnits=deg  UpperLimitStiffness=1e4  UpperLimitStiffnessUnits=N*m/deg  UpperLimitDamping=10  UpperLimitDampingUnits=N*m/(deg/s)  UpperLimitTransitionRegionWidth=0.1  UpperLimitTransitionRegionWidthUnits=deg  PositionTargetSpecify=off  PositionTargetPriority=High  PositionTargetValue=0  PositionTargetValueUnits=deg  VelocityTargetSpecify=on  VelocityTargetPriority=High  VelocityTargetValue=hoverVel  VelocityTargetValueUnits=rad/s
  Outrunner Motor : sm_lib/Body Elements/Solid  InertiaType=CalculateFromGeometry  Mass=motorMass  MassUnits=kg  CenterOfMass=[0 0 0]  CenterOfMassUnits=m  MomentsOfInertia=[1 1 1]  MomentsOfInertiaUnits=kg*m^2  ProductsOfInertia=[0 0 0]  ProductsOfInertiaUnits=kg*m^2  BasedOnType=Mass  Density=1000  DensityUnits=kg/(m^3)  DoExposeReferenceFrame=on  SerializedFrames=<Frames/>  GraphicType=FromGeometry  MarkerShape=Sphere  MarkerSize=10  MarkerSizeUnits=m  GraphicVisPropType=SimpleVisualProperties  GraphicDiffuseColor=[0.6 0.0 0.2]  GraphicSpecularColor=[0.5 0.5 0.5 1.0]  GraphicAmbientColor=[0.15 0.15 0.15 1.0]  GraphicEmissiveColor=[0.0 0.0 0.0 1.0]  GraphicShininess=75  GraphicOpacity=1.0  GeometryShape=Cylinder  RectangleSize=[1 1]  RectangleSizeUnits=m  BrickDimensions=[1 1 0.01]  BrickDimensionUnits=m  CylinderRadius=0.02  CylinderRadiusUnits=m  CylinderLength=0.05  CylinderLengthUnits=m  SphereRadius=1  SphereRadiusUnits=m  EllipsoidRadii=[1 1 1]  EllipsoidRadiiUnits=m  ExtrusionCrossSection=[1 1; -1 1; -1 -1; 1 -1]  ExtrusionCrossSectionUnits=m  ExtrusionLength=1  ExtrusionLengthUnits=m  PolygonNumSides=3  PolygonOuterRadius=1  PolygonOuterRadiusUnits=m  ExtGeomFileType=STL  ExtGeomFileUnits=m  RevolutionCrossSection=[1 1; 1 -1; 2 -1; 2 1]  RevolutionCrossSectionUnits=m  RevolutionExtent=Full  RevolutionAngle=180  RevolutionAngleUnits=deg
  PS-Simulink Converter3 : nesl_utility/PS-Simulink Converter  PhysicalDomain=network_engine_domain  SubClassName=ps_output  LeftPortType=input  RightPortType=output  PseudoPeriodic=off  Frequencies=[]  Unit=1  AffineConversion=off
  Product{1..4} (4 alike) : Product
  Propeller : sm_lib/Body Elements/Solid  InertiaType=CalculateFromGeometry  Mass=propellerMass  MassUnits=kg  CenterOfMass=[0 0 0]  CenterOfMassUnits=m  MomentsOfInertia=[1 1 1]  MomentsOfInertiaUnits=kg*m^2  ProductsOfInertia=[0 0 0]  ProductsOfInertiaUnits=kg*m^2  BasedOnType=Mass  Density=1000  DensityUnits=kg/(m^3)  DoExposeReferenceFrame=on  SerializedFrames=<Frames/>  GraphicType=FromGeometry  MarkerShape=Sphere  MarkerSize=10  MarkerSizeUnits=m  GraphicVisPropType=SimpleVisualProperties  GraphicDiffuseColor=[0.6 0.0 0.2]  GraphicSpecularColor=[0.5 0.5 0.5 1.0]  GraphicAmbientColor=[0.15 0.15 0.15 1.0]  GraphicEmissiveColor=[0.0 0.0 0.0 1.0]  GraphicShininess=75  GraphicOpacity=1.0  GeometryShape=Brick  RectangleSize=[1 1]  RectangleSizeUnits=m  BrickDimensions=[0.2 0.03 0.01]  BrickDimensionUnits=m  CylinderRadius=0.02  CylinderRadiusUnits=m  CylinderLength=0.05  CylinderLengthUnits=m  SphereRadius=1  SphereRadiusUnits=m  EllipsoidRadii=[1 1 1]  EllipsoidRadiiUnits=m  ExtrusionCrossSection=[1 1; -1 1; -1 -1; 1 -1]  ExtrusionCrossSectionUnits=m  ExtrusionLength=1  ExtrusionLengthUnits=m  PolygonNumSides=3  PolygonOuterRadius=1  PolygonOuterRadiusUnits=m  ExtGeomFileType=STL  ExtGeomFileUnits=m  RevolutionCrossSection=[1 1; 1 -1; 2 -1; 2 1]  RevolutionCrossSectionUnits=m  RevolutionExtent=Full  RevolutionAngle=180  RevolutionAngleUnits=deg
  Rigid Transform1 : sm_lib/Frames and Transforms/Rigid Transform  TranslationMethod=Cartesian  TranslationStandardOffset=0  TranslationLengthUnit=m  TranslationStandardAxis=+Z  TranslationCartesianOffset=[0 0 0.03]  TranslationROffset=0  TranslationROffsetUnits=m  TranslationZOffset=0  TranslationZOffsetUnits=m  TranslationThetaOffset=0  TranslationThetaOffsetUnits=deg  RotationMethod=StandardAxis  RotationAngleUnits=deg  RotationStandardAxis=+Z  RotationAngle=0.0  RotationArbitraryAxis=[0 0 1]  FollAlignAxisA=+X  BaseAlignAxisA=+Y  FollAlignAxisB=+Y  BaseAlignAxisB=+Z  RotationSequenceAxes=FollowerAxes  RotationSequence=XYX  RotationSequenceAngles=[0 0 0]  RotationSequenceAnglesUnits=deg  RotationMatrix=[1 0 0; 0 1 0; 0 0 1]
  Simulink-PS Converter1 : nesl_utility/Simulink-PS Converter  PhysicalDomain=network_engine_domain  SubClassName=ps_input  LeftPortType=input  RightPortType=output  PseudoPeriodic=off  Frequencies=[]  NoiseDistribution=none  NoiseParameters=[]  Unit=1  AffineConversion=off  FilteringAndDerivatives=zero  SimscapeFilterOrder=1  InputFilterTimeConstant=0.001  UdotUserProvided=1
  Simulink-PS Converter2 : nesl_utility/Simulink-PS Converter  PhysicalDomain=network_engine_domain  SubClassName=ps_input  LeftPortType=input  RightPortType=output  PseudoPeriodic=off  Frequencies=[]  NoiseDistribution=none  NoiseParameters=[]  Unit=1  AffineConversion=off  FilteringAndDerivatives=zero  SimscapeFilterOrder=1  InputFilterTimeConstant=0.001  UdotUserProvided=1
  Sum : Sum  Inputs=|+-
  Sum2 : Sum  Inputs=|+-
  drag_konstant : Gain  Gain=KDrag
  motor_konstant : Constant  Value=Km
  rad/s to RPM : Gain  Gain=60/2/pi
  trust_konstant : Gain  Gain=Ktrust
  pos : PMIOPort  Side=Left
  RPM : Outport
  trust : Outport  Port=2
  wires:
  Product4/1 -> trust_konstant/1
  CV_CCV/1 -> Product4/1, Product3/1
  Product3/1 -> Sum/1
  volt/1 -> Product3/2
  drag_konstant/1 -> Sum2/2
  Sum2/1 -> Simulink-PS Converter2/1
  PS-Simulink Converter3/1 -> Product4/2, Product1/1, rad/s to RPM/1, drag_konstant/1
  Sum/1 -> Ankrmodstand/1
  Ankrmodstand/1 -> Product2/1  "motor current"
  Product2/1 -> Sum2/1  "motor torque"
  trust_konstant/1 -> Simulink-PS Converter1/1, trust/1
  Product1/1 -> Sum/2
  motor_konstant/1 -> Product1/2, Product2/2
  rad/s to RPM/1 -> RPM/1
  connections:
  Rigid Transform1/RConn1 -- External Force and Torque/RConn1 -- Propeller/RConn1
  Outrunner Motor/RConn1 -- pos/RConn1 -- Motor axle/LConn1
  Simulink-PS Converter2/RConn1 -- Motor axle/LConn2
  Motor axle/RConn1 -- Rigid Transform1/LConn1
  Motor axle/RConn2 -- PS-Simulink Converter3/LConn1
  Simulink-PS Converter1/RConn1 -- External Force and Torque/LConn1
